simulink model "JetSki_Ver2"  (R2017a)
settings: Solver=ode4  StartTime=0.0  StopTime=28  FixedStep=0.005  RelTol=1e-3
values from neighbouring files (symbols this model uses):
  acceptanceR = 10    [initParameters.m]    (also in scenario1_uF5ms_DeltaF10.mat; scenario1_uF5ms_DeltaF10_LOS.mat; scenario1_uF5ms_DeltaF25.mat; scenario1_uF5ms_DeltaF25_LOS.mat)
  Aref = [0 1; -omega0^2 -2*damping*omega0]    [refSmoother.m]    (also in scenario1_uF5ms_DeltaF10.mat = [0  1; -6.25  -5]; scenario1_uF5ms_DeltaF10_LOS.mat = [0  1; -6.25  -5]; scenario1_uF5ms_DeltaF25.mat = [0  1; -6.25  -5]; scenario1_uF5ms_DeltaF25_LOS.mat = [0  1; -6.25  -5])
  Bref = [0 ; omega0^2]    [refSmoother.m]    (also in scenario1_uF5ms_DeltaF10.mat = [0 6.25]; scenario1_uF5ms_DeltaF10_LOS.mat = [0 6.25]; scenario1_uF5ms_DeltaF25.mat = [0 6.25]; scenario1_uF5ms_DeltaF25_LOS.mat = [0 6.25])
  craftSpeedCurvatureLookup = [0,1000 ... (first row only)    [CreateLookUpTableSpeedCurvature.m]    (also in scenario1_uF5ms_DeltaF10.mat = [0 1 2 3 4 5 6 7 8 9 10 12.5 ... (34 elements, 17x2)]; scenario1_uF5ms_DeltaF10_LOS.mat = [0 1 2 3 4 5 6 7 8 9 10 12.5 ... (34 elements, 17x2)]; scenario1_uF5ms_DeltaF25.mat = [0 1 2 3 4 5 6 7 8 9 10 12.5 ... (34 elements, 17x2)]; scenario1_uF5ms_DeltaF25_LOS.mat = [0 1 2 3 4 5 6 7 8 9 10 12.5 ... (34 elements, 17x2)])
  CTRL = Kc*LC1*LC2    [ControllerDesign.m]
  K = 2.06    [ControllerDesign.m]    (also in LookaheadBasedSteeringWithDynamicsAndBigTurn.m; initParameters.m; scenario1_uF5ms_DeltaF10.mat; scenario1_uF5ms_DeltaF10_LOS.mat)
  ki = 0.1/lookAheadDistance    (= 0.1)    [LookaheadBasedSteering.m]    (also in LookaheadBasedSteeringWithDynamicsAndBigTurn.m; initParameters.m = 0.01; scenario1_uF5ms_DeltaF10.mat = 0.004; scenario1_uF5ms_DeltaF10_LOS.mat = 0.004)
  kp = 1/lookAheadDistance    (= 1)    [LookaheadBasedSteeringWithDynamicsAndBigTurn.m]    (also in initParameters.m = 0.1; scenario1_uF5ms_DeltaF10.mat = 0.04; scenario1_uF5ms_DeltaF10_LOS.mat = 0.04; scenario1_uF5ms_DeltaF25.mat = 0.04)
  L = 3.25    [initParameters.m]
  lookAheadDistance = 1    [LookaheadBasedSteering.m]    (also in LookaheadBasedSteeringWithDynamics.m; LookaheadBasedSteeringWithDynamicsAndBigTurn.m; initParameters.m = 10; scenario1_uF5ms_DeltaF10.mat = 10.2034887623)
  obstacleList = [50, -5, 1,  pi-atan2(-5,50),15,15]    [initParameters.m]    (also in scenario1_uF5ms_DeltaF10.mat = [50 -5 1 3.24126130608 15 15]; scenario1_uF5ms_DeltaF10_LOS.mat = [50 -5 1 3.24126130608 15 15]; scenario1_uF5ms_DeltaF25.mat = [50 -5 1 3.24126130608 15 15]; scenario1_uF5ms_DeltaF25_LOS.mat = [50 -5 1 3.24126130608 15 15])
  pathCurvature = [0.000387339669156 0.000387339669156 0.000435861398373 0.00038761984579 0.000403869239907 0.000387905738489 0.000396085688617 0.000396234359996 0.00041940549491 0.00041001020904 0.000420199371031 0.000424770907578 ... (1135 elements, 1135x1)]    [scenario1_uF5ms_DeltaF10.mat]    (also in scenario1_uF5ms_DeltaF10_LOS.mat; scenario1_uF5ms_DeltaF25.mat; scenario1_uF5ms_DeltaF25_LOS.mat; scenario1_uF5ms_DeltaV25.mat)
  phiBeta = 0    [initParameters.m]    (also in scenario1_uF5ms_DeltaF10.mat; scenario1_uF5ms_DeltaF10_LOS.mat; scenario1_uF5ms_DeltaF25.mat; scenario1_uF5ms_DeltaF25_LOS.mat)
  Psi0 = 0    [initParameters.m]    (also in mainScript.m = craft.heading; scenario1_uF5ms_DeltaF10.mat; scenario1_uF5ms_DeltaF10_LOS.mat; scenario1_uF5ms_DeltaF25.mat)
  target = [100,0]    [initParameters.m]    (also in scenario1_uF5ms_DeltaF10.mat = [100 0]; scenario1_uF5ms_DeltaF10_LOS.mat = [100 0]; scenario1_uF5ms_DeltaF25.mat = [100 0]; scenario1_uF5ms_DeltaF25_LOS.mat = [100 0])
  Tdelta = 0.33    [LookaheadBasedSteeringWithDynamicsAndBigTurn.m]    (also in initParameters.m = 0.32; scenario1_uF5ms_DeltaF10.mat = 0.32; scenario1_uF5ms_DeltaF10_LOS.mat = 0.32; scenario1_uF5ms_DeltaF25.mat = 0.32)
  Tr = 1.72    [initParameters.m]    (also in scenario1_uF5ms_DeltaF10.mat; scenario1_uF5ms_DeltaF10_LOS.mat; scenario1_uF5ms_DeltaF25.mat; scenario1_uF5ms_DeltaF25_LOS.mat)
  u_craft = 5    [initParameters.m]    (also in scenario1_uF5ms_DeltaF10.mat; scenario1_uF5ms_DeltaF10_LOS.mat; scenario1_uF5ms_DeltaF25.mat; scenario1_uF5ms_DeltaF25_LOS.mat)
  v_current = 0    [initParameters.m]    (also in scenario1_uF5ms_DeltaF10.mat; scenario1_uF5ms_DeltaF10_LOS.mat; scenario1_uF5ms_DeltaF25.mat; scenario1_uF5ms_DeltaF25_LOS.mat)
  x0 = 0    [initParameters.m]    (also in lookAheadPathFollower.m = states(j,1); lookAheadPathFollowerD.m = states(j,1); mainScript.m = craft.pos.x; mmstream2arr.m = dxy(end,1))
  y0 = 0    [initParameters.m]    (also in lookAheadPathFollower.m = states(j,2); lookAheadPathFollowerD.m = states(j,2); mainScript.m = craft.pos.y; mmstream2arr.m = dxy(end,2))
libraries: simulink x1
settings Model: Creator=s120949  LastModifiedBy=Max
settings DataIOCC: SaveFormat=Array
settings OptimizationCC: BlockReduction=off  BooleanDataType=off  LifeSpan=inf
settings DebuggingCC: ReadBeforeWriteMsg=DisableAll  WriteAfterWriteMsg=DisableAll  WriteAfterReadMsg=DisableAll  SaveWithParameterizedLinksMsg=none  MultiTaskDSMMsg=none  SFUnexpectedBacktrackingDiag=warning  SFNoUnconditionalDefaultTransitionDiag=warning  SFExecutionAtInitializationDiag=none
settings HardwareCC: ProdBitPerPointer=32  ProdBitPerSizeT=32  ProdBitPerPtrDiffT=32  ProdLargestAtomicFloat=None  ProdIntDivRoundTo=Undefined  ProdEndianess=Unspecified  ProdWordSize=32  ProdHWDeviceType=32-bit Generic  TargetBitPerPointer=64  TargetBitPerSizeT=64  TargetBitPerPtrDiffT=64  TargetLongLongMode=on  TargetIntDivRoundTo=Zero  TargetEndianess=LittleEndian  TargetWordSize=64  TargetHWDeviceType=MATLAB Host  ProdEqTarget=off
settings ModelReferenceCC: PropagateSignalLabelsOutOfModel=off
settings SFSimCC: SFSimEcho=off
settings GRTTargetCC: TargetLangStandard=C89/C90 (ANSI)  GeneratePreprocessorConditionals=Disable all
settings ConfigComp: CovMetricSettings=dw  CovHtmlReporting=on  CovSaveCumulativeToWorkspaceVar=on  CovSaveSingleToWorkspaceVar=on  CovExternalEMLEnable=off  CovSFcnEnable=off

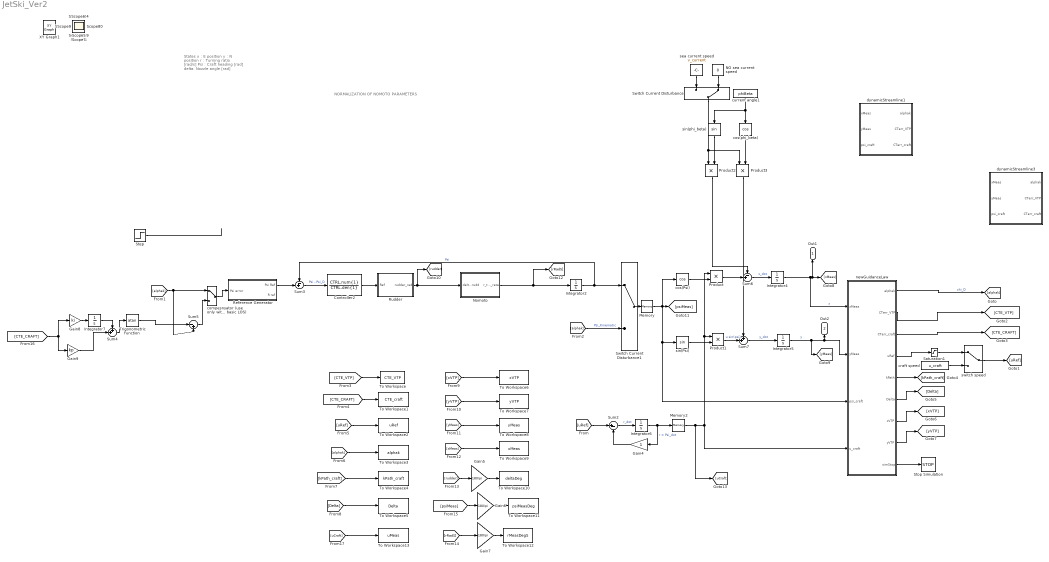
== system JetSki_Ver2 ==
  note: NORMALIZATION OF
      | NOMOTO PARAMETERS
  note: States
      | x : E position
      | y : N position
      | r : Turning ratio [rad/s]
      | Psi : Craft heading [rad]
      | delta: Nozzle angle [rad]
  Controller2 : TransferFcn  Numerator=CTRL.num{1}  Denominator=CTRL.den{1}
  Gain4 : Gain
  Gain5 : Gain  Gain=180/pi
  Gain6 : Gain  Gain=180/pi
  Gain7 : Gain  Gain=180/pi
  Gain8 : Gain  Gain=ki
  Gain9 : Gain  Gain=kp
  Integrator2 : Integrator  Priority=3  InitialCondition=Psi0  ContinuousStateAttributes='craft_Psi'
  Integrator4 : Integrator  Priority=1  InitialCondition=x0  ContinuousStateAttributes='craft_x'
  Integrator5 : Integrator  Priority=2  InitialCondition=y0  ContinuousStateAttributes='craft_y'
  Integrator6 : Integrator  Priority=4  InitialCondition=u_craft  ContinuousStateAttributes='craft_u'
  Integrator7 : Integrator  Priority=4  ContinuousStateAttributes='craft_r'
  Memory : Memory  X0=Psi0  InheritSampleTime=on
  Memory2 : Memory  X0=u_craft  InheritSampleTime=on
  NO sea current speed : Constant  Value=0
  Nomoto : Subsystem
  Product{,1..3} (4 alike) : Product
  Reference Generator : Subsystem
  Rudder : Subsystem
  Saturation1 : Saturate  UpperLimit=10  LowerLimit=0
  Step : Step  Time=3  After=pi  SampleTime=0
  Stop Simulation : Stop
  Sum2 : Sum  Inputs=|+-
  Sum3 : Sum  Inputs=-+|
  Sum4 : Sum  Inputs=++|
  Sum5 : Sum  Inputs=|-+
  Sum6 : Sum  Inputs=-+|
  Sum7 : Sum  Inputs=++|
  Switch Current Disturbance : ManualSwitch  CurrentSetting=0
  Switch Current Disturbance1 : ManualSwitch
  To Workspace : ToWorkspace  VariableName=CTE_VTP  SaveFormat=Structure With Time  SampleTime=-1
  To Workspace1 : ToWorkspace  VariableName=CTE_craft  SaveFormat=Structure With Time  SampleTime=-1
  To Workspace10 : ToWorkspace  VariableName=deltaDeg  SaveFormat=Structure With Time  SampleTime=-1
  To Workspace11 : ToWorkspace  VariableName=psiMeasDeg  SaveFormat=Structure With Time  SampleTime=-1
  To Workspace12 : ToWorkspace  VariableName=rMeasDegS  SaveFormat=Structure With Time  SampleTime=-1
  To Workspace13 : ToWorkspace  VariableName=uMeas  SaveFormat=Structure With Time  SampleTime=-1
  To Workspace2 : ToWorkspace  VariableName=uRef  SaveFormat=Structure With Time  SampleTime=-1
  To Workspace3 : ToWorkspace  VariableName=alphak  SaveFormat=Structure With Time  SampleTime=-1
  To Workspace4 : ToWorkspace  VariableName=kPath_craft  SaveFormat=Structure With Time  SampleTime=-1
  To Workspace5 : ToWorkspace  VariableName=Delta  SaveFormat=Structure With Time  SampleTime=-1
  To Workspace6 : ToWorkspace  VariableName=xVTP  SaveFormat=Structure With Time  SampleTime=-1
  To Workspace7 : ToWorkspace  VariableName=yVTP  SaveFormat=Structure With Time  SampleTime=-1
  To Workspace8 : ToWorkspace  VariableName=yMeas  SaveFormat=Structure With Time  SampleTime=-1
  To Workspace9 : ToWorkspace  VariableName=xMeas  SaveFormat=Structure With Time  SampleTime=-1
  Trigonometric Function : Trigonometry  Operator=atan
  compesnsator (use only with basic LOS) : ManualSwitch
  cos(Psi) : Trigonometry  Operator=cos
  cos(phi_beta) : Trigonometry  Operator=cos
  craft speed : Constant  Value=u_craft
  current angle1 : Constant  Value=phiBeta
  dynamicStreamline1 : MATLAB Function  TreatAsAtomicUnit=on
  dynamicStreamline3 : MATLAB Function  TreatAsAtomicUnit=on
  newGuidanceLaw : MATLAB Function  TreatAsAtomicUnit=on
  sea current speed : Constant  Value=v_current
  sin(Psi) : Trigonometry
  sin(phi_beta) : Trigonometry
  switch speed : ManualSwitch
  Out1 : Outport
  Out2 : Outport  Port=2
  Scope{,1..22,24..25} (25 alike) : Scope
  XY Graph1 : simulink/Sinks/XY Graph  IOType=viewer  xmin=-200  xmax=200  ymin=-200  ymax=200  st=-1
  wires:
  cos(Psi)/1 -> Product/2
  sin(Psi)/1 -> Product1/2
  Product1/1 -> Sum7/2  "u sin(psi)"
  Product/1 -> Sum6/2
  current angle1/1 -> sin(phi_beta)/1, cos(phi_beta)/1
  Switch Current Disturbance/1 -> Product2/1, Product3/1
  sin(phi_beta)/1 -> Product2/2
  cos(phi_beta)/1 -> Product3/2
  Product2/1 -> Sum6/1
  Product3/1 -> Sum7/1
  sea current speed/1 -> Switch Current Disturbance/1
  NO sea current speed/1 -> Switch Current Disturbance/2
  Sum6/1 -> Integrator4/1  "x_dot"
  Sum7/1 -> Integrator5/1  "y_dot"
  Integrator4/1 -> newGuidanceLaw/1(xMeas), [xMeas], Out1/1  "x"
  Integrator5/1 -> [yMeas], newGuidanceLaw/2(yMeas), Out2/1  "y"
  Sum3/1 -> Controller2/1  "Psi - Psi_D"
  Integrator2/1 -> Switch Current Disturbance1/1, Sum3/1  "Psi"
  Memory/1 -> [psiMeas], cos(Psi)/1, newGuidanceLaw/3(psi_craft), sin(Psi)/1
  Switch Current Disturbance1/1 -> Memory/1
  Reference Generator/1(Psi Ref) -> Sum3/2
  [uRef] -> Sum2/1
  newGuidanceLaw/1(alphak) -> [alphak]  "chi_D"
  [alphak] -> compesnsator (use only with basic LOS)/1, Sum5/2
  [alphak] -> Switch Current Disturbance1/2  "Psi_Kinematic"
  newGuidanceLaw/4(uRef) -> Saturation1/1
  Saturation1/1 -> switch speed/1
  switch speed/1 -> [uRef]
  craft speed/1 -> switch speed/2
  Memory2/1 -> [uCraft], newGuidanceLaw/4(u_craft), Product/1, Product1/1
  Gain4/1 -> Sum2/2
  Sum2/1 -> Integrator6/1  "r_dot"
  Integrator6/1 -> Memory2/1, Gain4/1  "r = Psi_dot"
  newGuidanceLaw/2(CTerr_VTP) -> [CTE_VTP]
  [CTE_VTP] -> To Workspace/1
  newGuidanceLaw/3(CTerr_craft) -> [CTE_CRAFT]
  [CTE_CRAFT] -> To Workspace1/1
  [uRef] -> To Workspace2/1
  [alphak] -> To Workspace3/1
  newGuidanceLaw/5(kPath) -> [kPath_craft]
  [kPath_craft] -> To Workspace4/1
  newGuidanceLaw/6(Delta) -> [Delta]
  [Delta] -> To Workspace5/1
  newGuidanceLaw/7(xVTP) -> [xVTP]
  newGuidanceLaw/8(yVTP) -> [yVTP]
  [xVTP] -> To Workspace6/1
  [yVTP] -> To Workspace7/1
  [yMeas] -> To Workspace8/1
  [xMeas] -> To Workspace9/1
  [rudder] -> Gain5/1
  Gain5/1 -> To Workspace10/1
  [psiMeas] -> Gain6/1
  Gain6/1 -> To Workspace11/1
  [rRadS] -> Gain7/1
  Gain7/1 -> To Workspace12/1
  newGuidanceLaw/9(simStop) -> Stop Simulation/1
  [CTE_CRAFT] -> Gain9/1, Gain8/1
  Gain8/1 -> Integrator7/1
  Gain9/1 -> Sum4/2
  Integrator7/1 -> Sum4/1
  Sum4/1 -> Trigonometric Function/1
  compesnsator (use only with basic LOS)/1 -> Reference Generator/1(Psi error)
  Trigonometric Function/1 -> Sum5/1
  Sum5/1 -> compesnsator (use only with basic LOS)/2
  [uCraft] -> To Workspace13/1
  Step/1 -> ?
  Rudder/1(rudder_rad) -> Nomoto/1(delta_rudd), [rudder]
  Controller2/1 -> Rudder/1(Ref)
  Nomoto/1(r_turning_rate) -> Integrator2/1, [rRadS]

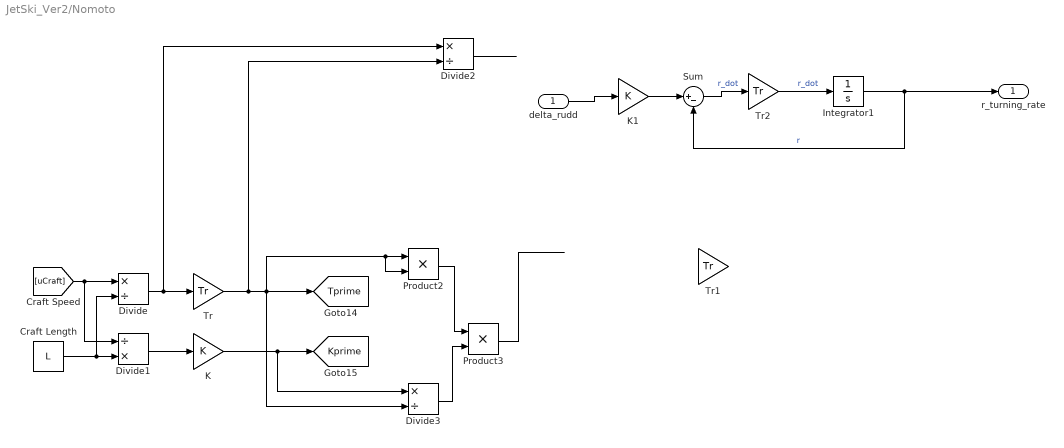
== system JetSki_Ver2/Nomoto ==
  delta_rudd : Inport
  Craft Length : Constant  Value=L
  Divide : Product  Inputs=*/
  Divide1 : Product  Inputs=/*
  Divide2 : Product  Inputs=*/
  Divide3 : Product  Inputs=*/
  Integrator1 : Integrator  Priority=4  ContinuousStateAttributes='craft_r'
  K : Gain  Gain=K
  K1 : Gain  Gain=K
  Product2 : Product
  Product3 : Product
  Sum : Sum  Inputs=|+-
  Tr : Gain  Gain=Tr
  Tr1 : Gain  Gain=Tr
  Tr2 : Gain  Gain=Tr
  r_turning_rate : Outport
  tag scope: Kprime=global, Tprime=global
  wires:
  delta_rudd/1 -> K1/1
  Integrator1/1 -> Sum/2, r_turning_rate/1  "r"
  Sum/1 -> Tr2/1  "r_dot"
  K1/1 -> Sum/1
  Tr2/1 -> Integrator1/1  "r_dot"
  [uCraft] -> Divide1/1, Divide/1
  Craft Length/1 -> Divide1/2, Divide/2
  Divide/1 -> Divide2/1, Tr/1
  Divide1/1 -> K/1
  Tr/1 -> Divide2/2, Product2/2, Product2/1, Divide3/2, [Tprime]
  K/1 -> Divide3/1, [Kprime]
  Divide2/1 -> ?
  Product2/1 -> Product3/1
  Divide3/1 -> Product3/2
  Product3/1 -> ?
  ? -> Tr1/1

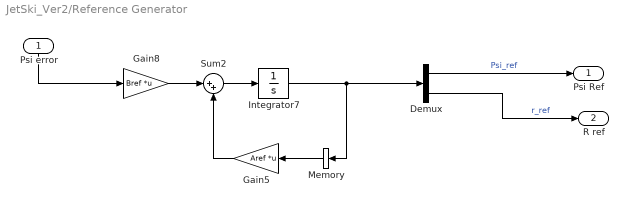
== system JetSki_Ver2/Reference Generator ==
  Psi error : Inport
  Demux : Demux  Outputs=2
  Gain5 : Gain  Gain=Aref  Multiplication=Matrix(K*u) (u vector)
  Gain8 : Gain  Gain=Bref  Multiplication=Matrix(K*u) (u vector)
  Integrator7 : Integrator  Priority=99  InitialCondition=[Psi0;0]  ContinuousStateAttributes='craft_r'
  Memory : Memory  InheritSampleTime=on
  Sum2 : Sum  Inputs=|++
  Psi Ref : Outport
  R ref : Outport  Port=2
  wires:
  Demux/1 -> Psi Ref/1  "Psi_ref"
  Gain8/1 -> Sum2/1
  Integrator7/1 -> Demux/1, Memory/1
  Gain5/1 -> Sum2/2
  Sum2/1 -> Integrator7/1
  Demux/2 -> R ref/1  "r_ref"
  Psi error/1 -> Gain8/1
  Memory/1 -> Gain5/1

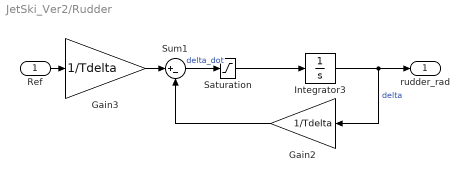
== system JetSki_Ver2/Rudder ==
  Ref : Inport
  Gain2 : Gain  Gain=1/Tdelta
  Gain3 : Gain  Gain=1/Tdelta
  Integrator3 : Integrator  Priority=5  LimitOutput=on  UpperSaturationLimit=0.26  LowerSaturationLimit=-0.26  ContinuousStateAttributes='craft_delta'
  Saturation : Saturate  UpperLimit=0.5236  LowerLimit=-0.5236
  Sum1 : Sum  Inputs=|+-
  rudder_rad : Outport
  wires:
  Gain3/1 -> Sum1/1
  Sum1/1 -> Saturation/1  "delta_dot"
  Gain2/1 -> Sum1/2
  Integrator3/1 -> rudder_rad/1, Gain2/1  "delta"
  Saturation/1 -> Integrator3/1
  Ref/1 -> Gain3/1

== matlab function JetSki_Ver2/dynamicStreamline3 ==
  data: alphak output double; xMeas input; yMeas input; obstacleList parameter; target parameter; CTerr_VTP output; lookAheadDistance parameter; acceptanceR parameter; psi_craft input; u_craft parameter; CTerr_craft output
function [alphak,CTerr_VTP, CTerr_craft] = fcn(xMeas, yMeas, obstacleList, target, lookAheadDistance, acceptanceR, psi_craft, u_craft)
coder.extrinsic('tic');
coder.extrinsic('toc');
coder.extrinsic('evalin');
coder.extrinsic('disp');
coder.extrinsic('get_param');
coder.extrinsic('strcat');
coder.extrinsic('num2str');
coder.extrinsic('assignin');

persistent trajectory trajX trajY trigger calculated tanCurve prevAlphaK turnCounter
waypoint = 0;
% deal with missing data
if isempty(trigger)
    trigger = obstacleList(:,3);
end;
if isempty(calculated)
    calculated = obstacleList(:,3);
end;

if isempty(trajectory)
    tx = target(1);
    ty = target(2);
    [trajX,trajY] = getTrajectory(0, 0, tx,ty, obstacleList);
end
if isempty(tanCurve)
        tanCurve = atan2(trajY,trajX);
end
if isempty(prevAlphaK)
    prevAlphaK = 0;
end
if isempty(turnCounter)
    turnCounter = 0;
end

xT = trajX(1);
yT = trajY(1);
%PsiWpts = atan2(yT-yMeas, xT-xMeas);

% Create Virtual Target ahead
pointAhead = [xMeas+lookAheadDistance*cos(psi_craft),yMeas+lookAheadDistance*sin(psi_craft)];

% Check cross track error between VTP and path
dx = trajX - pointAhead(1);
dy = trajY - pointAhead(2);
[CTerr_VTP, ind_VTP] = min(hypot(dx, dy));

% Find out if the VPT is on one side or the other
angle1 = atan2(trajY(ind_VTP)-trajY(1),trajX(ind_VTP)-trajX(1));
angle2 = atan2(pointAhead(2)-trajY(1),pointAhead(1)-trajX(1));
if (angle2<angle1) % Craft inside the curve
   CTerr_VTP = -CTerr_VTP;
end

% Obtain heading reference (it is the projection of the VTP on the path)
alphak = atan2(trajY(ind_VTP)-yMeas,trajX(ind_VTP)-xMeas);


% Check cross track error between craft and path
dx = trajX - xMeas;
dy = trajY - yMeas;
[CTerr_craft, ind] = min(hypot(dx, dy));

% Find out if the craft is on one side or the other
angle1 = atan2(trajY(ind)-trajY(1),trajX(ind)-trajX(1));
angle2 = atan2(yMeas-trajY(1),xMeas-trajX(1));
if (angle2<angle1) % Craft inside the curve
    CTerr_craft = -CTerr_craft;
end

%% Alternative (traditional LOS) the particle is on the tangent of the path

craftProjection = [trajX(ind),trajY(ind)];
angleTangent = tanCurve(ind);
pLOS = [craftProjection(1)+lookAheadDistance*cos(angleTangent),craftProjection(2)+lookAheadDistance*sin(angleTangent)];

alphak = atan2(pLOS(2)-yMeas,pLOS(1)-xMeas);
alphak = alphak - turnCounter*2*pi;
%% Correct angle

if ((abs(prevAlphaK-alphak)>pi)) % a tan discontinuity happened
    if (alphak>prevAlphaK)   
         alphak = alphak - 2*pi;
         turnCounter = turnCounter + 1;
    else
         alphak = alphak + 2*pi;
         turnCounter = turnCounter - 1;
    end;
        
end
   
prevAlphaK = alphak;
end

== matlab function JetSki_Ver2/dynamicStreamline1 ==
  data: alphak output double; xMeas input; yMeas input; obstacleList parameter; target parameter; CTerr_VTP output; lookAheadDistance parameter; acceptanceR parameter; psi_craft input; u_craft parameter; CTerr_craft output
function [alphak,CTerr_VTP, CTerr_craft] = fcn(xMeas, yMeas, obstacleList, target, lookAheadDistance, acceptanceR, psi_craft, u_craft)
coder.extrinsic('tic');
coder.extrinsic('toc');
coder.extrinsic('evalin');
coder.extrinsic('disp');
coder.extrinsic('get_param');
coder.extrinsic('strcat');
coder.extrinsic('num2str');
coder.extrinsic('assignin');

persistent trajectory trajX trajY trigger calculated tanCurve prevAlphaK turnCounter
waypoint = 0;
% deal with missing data
if isempty(trigger)
    trigger = obstacleList(:,3);
end;
if isempty(calculated)
    calculated = obstacleList(:,3);
end;

if isempty(trajectory)
    tx = target(1);
    ty = target(2);
    [trajX,trajY] = getTrajectory(0, 0, tx,ty, obstacleList);
end
if isempty(tanCurve)
        tanCurve = atan2(trajY,trajX);
end
if isempty(prevAlphaK)
    prevAlphaK = 0;
end
if isempty(turnCounter)
    turnCounter = 0;
end

xT = trajX(1);
yT = trajY(1);
%PsiWpts = atan2(yT-yMeas, xT-xMeas);

% Create Virtual Target ahead
pointAhead = [xMeas+lookAheadDistance*cos(psi_craft),yMeas+lookAheadDistance*sin(psi_craft)];

% Check cross track error between VTP and path
dx = trajX - pointAhead(1);
dy = trajY - pointAhead(2);
[CTerr_VTP, ind_VTP] = min(hypot(dx, dy));

% Find out if the VPT is on one side or the other
angle1 = atan2(trajY(ind_VTP)-trajY(1),trajX(ind_VTP)-trajX(1));
angle2 = atan2(pointAhead(2)-trajY(1),pointAhead(1)-trajX(1));
if (angle2<angle1) % Craft inside the curve
   CTerr_VTP = -CTerr_VTP;
end

% Obtain heading reference (it is the projection of the VTP on the path)
alphak = atan2(trajY(ind_VTP)-yMeas,trajX(ind_VTP)-xMeas);


% Check cross track error between craft and path
dx = trajX - xMeas;
dy = trajY - yMeas;
[CTerr_craft, ind] = min(hypot(dx, dy));

% Find out if the craft is on one side or the other
angle1 = atan2(trajY(ind)-trajY(1),trajX(ind)-trajX(1));
angle2 = atan2(yMeas-trajY(1),xMeas-trajX(1));
if (angle2<angle1) % Craft inside the curve
    CTerr_craft = -CTerr_craft;
end

%% Alternative (traditional LOS) the particle is on the tangent of the path

craftProjection = [trajX(ind),trajY(ind)];
angleTangent = tanCurve(ind);
pLOS = [craftProjection(1)+lookAheadDistance*cos(angleTangent),craftProjection(2)+lookAheadDistance*sin(angleTangent)];

alphak = atan2(pLOS(2)-yMeas,pLOS(1)-xMeas);
alphak = alphak - turnCounter*2*pi;
%% Correct angle

if ((abs(prevAlphaK-alphak)>pi)) % a tan discontinuity happened
    if (alphak>prevAlphaK)   
         alphak = alphak - 2*pi;
         turnCounter = turnCounter + 1;
    else
         alphak = alphak + 2*pi;
         turnCounter = turnCounter - 1;
    end;
        
end
   
prevAlphaK = alphak;
end

== matlab function JetSki_Ver2/newGuidanceLaw ==
  data: alphak output double; xMeas input; yMeas input; obstacleList parameter; target parameter; CTerr_VTP output; lookAheadDistance parameter; pathCurvature parameter; acceptanceR parameter; craftSpeedCurvatureLookup parameter; psi_craft input; u_craft input; CTerr_craft output; uRef output; kPath output; Delta output; xVTP output; yVTP output; simStop output
function [alphak,CTerr_VTP, CTerr_craft, uRef, kPath, Delta, xVTP, yVTP, simStop] = fcn(xMeas, yMeas, obstacleList, target, lookAheadDistance, pathCurvature, acceptanceR, craftSpeedCurvatureLookup, psi_craft, u_craft)
coder.extrinsic('tic');
coder.extrinsic('toc');
coder.extrinsic('evalin');
coder.extrinsic('disp');
coder.extrinsic('get_param');
coder.extrinsic('strcat');
coder.extrinsic('num2str');
coder.extrinsic('assignin');

%% 17/02/15 - attempt to implement variable lookahead reference from curvature
% attempt to add variable speed control from curvature

persistent trajectory trajX trajY trigger calculated tanCurve prevAlphaK turnCounter lookAheadDistanceP baseLookAheadDistance

% deal with missing data
if isempty(trigger)
    trigger = obstacleList(:,3);
end;

%if isempty(baseLookAheadDistance)
    baseLookAheadDistance = 25;
%end;

if isempty(lookAheadDistanceP)
    lookAheadDistanceP = 0;
end;

if isempty(calculated)
    calculated = obstacleList(:,3);
end;

if isempty(trajectory)
    tx = target(1);
    ty = target(2);
    [trajX,trajY] = getTrajectory(0, 0, tx,ty, obstacleList);
    trajectory = [trajX, trajY];
end

% if isempty(pathCurvature)
%     pathCurvature = CurvatureEstimation(trajectory); % NOT SUPPORTED IN
%     CODE GENERATION, USE ALTERNATIVE FUNCTION TO GET CURVATURE, FOR NOW
%     IT IS JUST PRECOMPUTED BEFORE RUNNING
% end

if isempty(tanCurve)
        tanCurve = atan2(trajY,trajX);
end

if isempty(prevAlphaK)
    prevAlphaK = 0;
end

if isempty(turnCounter)
    turnCounter = 0;
end


% Check cross track error between craft and path
dx = trajX - xMeas;
dy = trajY - yMeas;
[CTerr_craft, ind_craft] = min(hypot(dx, dy));


% Create Virtual Target ahead (first case to check the curvature)
VTP = [xMeas+lookAheadDistance*cos(psi_craft), yMeas+lookAheadDistance*sin(psi_craft)];
xVTP = VTP(1);
yVTP = VTP(2);



% Check cross track error between VTP and path
dx = trajX - VTP(1);
dy = trajY - VTP(2);
[~, ind_VTP] = min(hypot(dx, dy));

% Redraw particle according to curvature
lookAheadDistance = baseLookAheadDistance - 650*max(pathCurvature(ind_VTP),pathCurvature(ind_craft));
if (lookAheadDistance<5)
    lookAheadDistance = 5;
end;
if isnan(lookAheadDistance)
    lookAheadDistance = baseLookAheadDistance;
end;
Delta = lookAheadDistance;
VTP = [xMeas+Delta*cos(psi_craft),yMeas+Delta*sin(psi_craft)];
xVTP = VTP(1);
yVTP = VTP(2);
% Check cross track error between new VTP and path
dx = trajX - VTP(1);
dy = trajY - VTP(2);
[CTerr_VTP, ind_VTP] = min(hypot(dx, dy));
VTP_projection = [trajX(ind_VTP),trajY(ind_VTP)];

% angleTangent = tanCurve(ind_VTP);
% pLOS = [VTP_projection(1)+lookAheadDistanceP*cos(angleTangent),VTP_projection(2)+lookAheadDistanceP*sin(angleTangent)];

% Reference angle is the vector that points from the craft to the
% projection of the VTP on the track
alphak = atan2(VTP_projection(2)-yMeas,VTP_projection(1)-xMeas);



% Calculate cross-track errors
% Find out if the craft is on one side or the other
angle1 = atan2(trajY(ind_craft)-trajY(1),trajX(ind_craft)-trajX(1));
angle2 = atan2(yMeas-trajY(1),xMeas-trajX(1));
if (angle2<angle1) % Craft inside the curve
    CTerr_craft = -CTerr_craft;
end

% Find out if the VPT is on one side or the other
angle1 = atan2(trajY(ind_VTP)-trajY(1),trajX(ind_VTP)-trajX(1));
angle2 = atan2(VTP(2)-trajY(1),VTP(1)-trajX(1));
if (angle2<angle1) % Craft inside the curve
   CTerr_VTP = -CTerr_VTP;
end

%% Alternative (traditional LOS) the particle is on the tangent of the path

% craftProjection = [trajX(ind_craft),trajY(ind_craft)];
% angleTangent = tanCurve(ind_craft);
% pLOS = [craftProjection(1)+lookAheadDistance*cos(angleTangent),craftProjection(2)+lookAheadDistance*sin(angleTangent)];

% alphak = atan2(pLOS(2)-yMeas,pLOS(1)-xMeas);
% alphak = alphak - turnCounter*2*pi;
%% Correct angle jumps (TODO: CHECK properly)

if ((abs(prevAlphaK-alphak)>pi)) % a tan discontinuity happened
    if (alphak>prevAlphaK)   
         alphak = alphak - 2*pi;
         turnCounter = turnCounter + 1;
    else
         alphak = alphak + 2*pi;
         turnCounter = turnCounter - 1;
    end;
        
end
   
prevAlphaK = alphak;

% Curvature -> speed reference, it takes the maximum curvature between the
% craft and the particle (conservative)
maxCurvature = max(pathCurvature(ind_craft),pathCurvature(ind_VTP)); 
uRef = interp1(craftSpeedCurvatureLookup(:,2),craftSpeedCurvatureLookup(:,1),maxCurvature);
kPath = pathCurvature(ind_craft);


simStop = 0;
if (xMeas>100)
    simStop = 1;
end
end
